simulink subsystem "cvrs_heart_cycle"  (R2020b)
settings: Solver=VariableStepAuto  StartTime=0.0  StopTime=10.0  RelTol=1e-3
settings Model: Creator=RH  LastModifiedBy=Marco

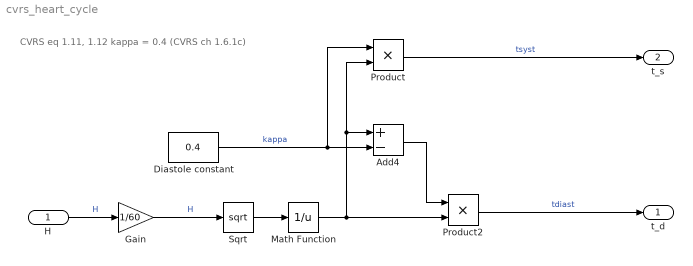
== system cvrs_heart_cycle ==
  note: CVRS eq 1.11, 1.12
      | kappa = 0.4 (CVRS ch 1.6.1c)
  H : Inport  Unit=1/min
  Add4 : Sum  Inputs=+-
  Diastole constant : Constant  Value=0.4
  Gain : Gain  Gain=1/60
  Math Function : Math  Operator=reciprocal  SaturateOnIntegerOverflow=on
  Product : Product
  Product2 : Product
  Sqrt : Sqrt  SaturateOnIntegerOverflow=on
  t_d : Outport  Unit=s
  t_s : Outport  Port=2  Unit=s
  wires:
  Math Function/1 -> Product2/2, Add4/1, Product/2
  Diastole constant/1 -> Add4/2, Product/1  "kappa"
  Sqrt/1 -> Math Function/1
  Add4/1 -> Product2/1
  H/1 -> Gain/1  "H"
  Product/1 -> t_s/1  "tsyst"
  Product2/1 -> t_d/1  "tdiast"
  Gain/1 -> Sqrt/1  "H"
